simulink model "SF040A_MotVel"  (R2013b)
settings: Solver=FixedStepDiscrete  SolverMode=SingleTasking  StartTime=0.0  StopTime=1  FixedStep=6.25E-5  RelTol=1e-3
undefined symbols (not defined in the file or in its folder): ARCHGLBPRM_2MILLISEC_SEC_F32, ARCHGLBPRM_2PI_ULS_F32, ARCHGLBPRM_FLOATZEROTHD_ULS_F32, ARCHGLBPRM_PI_ULS_F32, BITMASK16BIT_CNT_U32, BUFSIZE_CNT_U08, BUFSIZECOMBD_CNT_U08, MOTAGMECHIDPTSIGTHD_ULS_U08, MOTVELMAXININVAL_CNT_U08, SECTOMICROSEC_ULS_F32, ZEROTISTAMP_MICROSEC_F32, ZEROTISTAMP_MICROSEC_U32
libraries: simulink x7, NxtrLim x2, FixdToFloat x1
(part 2 of 2)

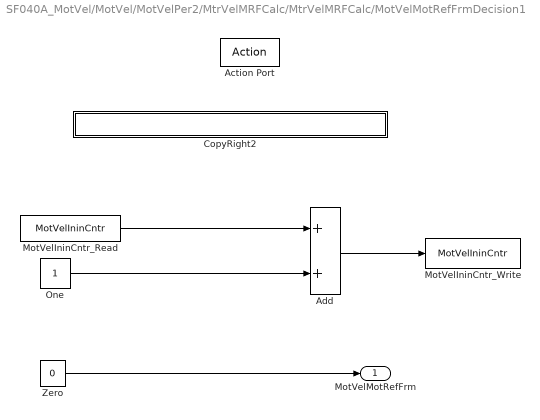
== system SF040A_MotVel/MotVel/MotVelPer2/MtrVelMRFCalc/MtrVelMRFCalc/MotVelMotRefFrmDecision1 ==
  Action Port : ActionPort  ActionType=then
  Add : Sum  OutDataTypeStr=Inherit: Inherit via back propagation
  CopyRight2 : Subsystem  Description=|  mask(Copyright Information){none=on}
      | Copyright info block.                                               
      |                                                                     
      | Place copyright information at the top of every subsystem in design.
      mask prompts: none "No parameters"
      mask help: Place copyright information at the top of every subsystem in design.
      mask Display:
      | NxtrConf = 'Nexteer Confidential';
      | 
      | sys = bdroot; %handle for the current model ("system")
      | first = get_param(sys,'Created');
      | first = first(end-3:end);  %year is last four digits
      | 
      | last = get_param(sys,'LastModifiedDate');
      | if isempty(last)
      |     last = datestr(now,'yyyy');
      | else
      |     last = last(end-3:end);
      | end
      | 
      | if strcmp(first,last)
      |     fprintf('%s -- Copyright %s Nexteer',NxtrConf,first)
      | else
      |     fprintf('%s -- %s%s- %s Nexteer',NxtrConf,char(169),first,last)
      | end
  MotVelIninCntr_Read : DataStoreRead  DataStoreName=MotVelIninCntr
  MotVelIninCntr_Write : DataStoreWrite  DataStoreName=MotVelIninCntr
  One : Constant  OutDataTypeStr=uint8
      settings: AttributesFormatString=%<OutDataTypeStr>
  Zero : Constant  Value=0  OutDataTypeStr=single
      settings: AttributesFormatString=%<OutDataTypeStr>
  MotVelMotRefFrm : Outport
  wires:
  Zero/1 -> MotVelMotRefFrm/1
  Add/1 -> MotVelIninCntr_Write/1
  One/1 -> Add/2
  MotVelIninCntr_Read/1 -> Add/1

== system SF040A_MotVel/MotVel/MotVelPer2/MtrVelMRFCalc/MtrVelMRFCalc/MotVelMotRefFrmDecision2 ==
  MotVelMrf : Inport
  Action Port : ActionPort  ActionType=else
  CopyRight2 : Subsystem  Description=|  mask(Copyright Information){none=on}
      | Copyright info block.                                               
      |                                                                     
      | Place copyright information at the top of every subsystem in design.
      mask prompts: none "No parameters"
      mask help: Place copyright information at the top of every subsystem in design.
      mask Display:
      | NxtrConf = 'Nexteer Confidential';
      | 
      | sys = bdroot; %handle for the current model ("system")
      | first = get_param(sys,'Created');
      | first = first(end-3:end);  %year is last four digits
      | 
      | last = get_param(sys,'LastModifiedDate');
      | if isempty(last)
      |     last = datestr(now,'yyyy');
      | else
      |     last = last(end-3:end);
      | end
      | 
      | if strcmp(first,last)
      |     fprintf('%s -- Copyright %s Nexteer',NxtrConf,first)
      | else
      |     fprintf('%s -- %s%s- %s Nexteer',NxtrConf,char(169),first,last)
      | end
  MotVelMotRefFrm : Outport
  wires:
  MotVelMrf/1 -> MotVelMotRefFrm/1

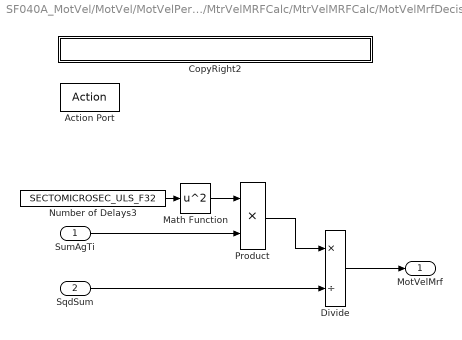
== system SF040A_MotVel/MotVel/MotVelPer2/MtrVelMRFCalc/MtrVelMRFCalc/MotVelMrfDecision1 ==
  SumAgTi : Inport
  SqdSum : Inport  Port=2
  Action Port : ActionPort  ActionType=then
  CopyRight2 : Subsystem  Description=|  mask(Copyright Information){none=on}
      | Copyright info block.                                               
      |                                                                     
      | Place copyright information at the top of every subsystem in design.
      mask prompts: none "No parameters"
      mask help: Place copyright information at the top of every subsystem in design.
      mask Display:
      | NxtrConf = 'Nexteer Confidential';
      | 
      | sys = bdroot; %handle for the current model ("system")
      | first = get_param(sys,'Created');
      | first = first(end-3:end);  %year is last four digits
      | 
      | last = get_param(sys,'LastModifiedDate');
      | if isempty(last)
      |     last = datestr(now,'yyyy');
      | else
      |     last = last(end-3:end);
      | end
      | 
      | if strcmp(first,last)
      |     fprintf('%s -- Copyright %s Nexteer',NxtrConf,first)
      | else
      |     fprintf('%s -- %s%s- %s Nexteer',NxtrConf,char(169),first,last)
      | end
  Divide : Product  Inputs=*/
  Math Function : Math  Operator=square  SaturateOnIntegerOverflow=on
  Number of Delays3 : Constant  Value=SECTOMICROSEC_ULS_F32
  Product : Product
  MotVelMrf : Outport
  wires:
  Number of Delays3/1 -> Math Function/1
  Math Function/1 -> Product/1
  SumAgTi/1 -> Product/2
  SqdSum/1 -> Divide/2
  Divide/1 -> MotVelMrf/1
  Product/1 -> Divide/1

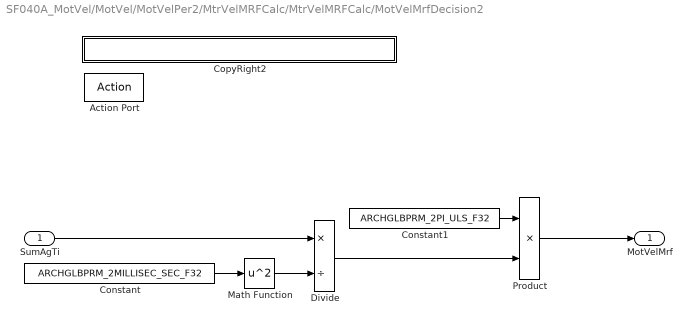
== system SF040A_MotVel/MotVel/MotVelPer2/MtrVelMRFCalc/MtrVelMRFCalc/MotVelMrfDecision2 ==
  SumAgTi : Inport
  Action Port : ActionPort  ActionType=else
  Constant : Constant  Value=ARCHGLBPRM_2MILLISEC_SEC_F32
  Constant1 : Constant  Value=ARCHGLBPRM_2PI_ULS_F32
  CopyRight2 : Subsystem  Description=|  mask(Copyright Information){none=on}
      | Copyright info block.                                               
      |                                                                     
      | Place copyright information at the top of every subsystem in design.
      mask prompts: none "No parameters"
      mask help: Place copyright information at the top of every subsystem in design.
      mask Display:
      | NxtrConf = 'Nexteer Confidential';
      | 
      | sys = bdroot; %handle for the current model ("system")
      | first = get_param(sys,'Created');
      | first = first(end-3:end);  %year is last four digits
      | 
      | last = get_param(sys,'LastModifiedDate');
      | if isempty(last)
      |     last = datestr(now,'yyyy');
      | else
      |     last = last(end-3:end);
      | end
      | 
      | if strcmp(first,last)
      |     fprintf('%s -- Copyright %s Nexteer',NxtrConf,first)
      | else
      |     fprintf('%s -- %s%s- %s Nexteer',NxtrConf,char(169),first,last)
      | end
  Divide : Product  Inputs=*/
  Math Function : Math  Operator=square  SaturateOnIntegerOverflow=on
  Product : Product
  MotVelMrf : Outport
  wires:
  SumAgTi/1 -> Divide/1
  Constant/1 -> Math Function/1
  Math Function/1 -> Divide/2
  Divide/1 -> Product/2
  Constant1/1 -> Product/1
  Product/1 -> MotVelMrf/1

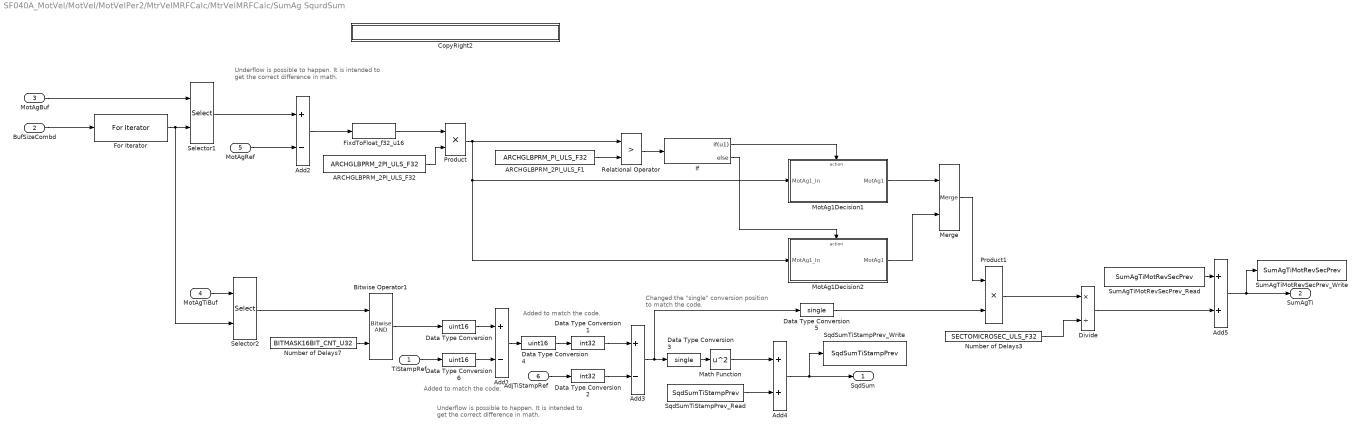
== system SF040A_MotVel/MotVel/MotVelPer2/MtrVelMRFCalc/MtrVelMRFCalc/SumAg SqurdSum ==
  note: Added to match the code.
  note: Underflow is possible to happen. It is intended
      | to get the correct difference in math.
  note: Underflow is possible to happen. It is intended
      | to get the correct difference in math.
  note: Changed the "single" conversion position
      |  to match the code.
  note: Added to match the code.
  TiStampRef : Inport
  BufSizeCombd : Inport  Port=2
  MotAgBuf : Inport  Port=3
  MotAgTiBuf : Inport  Port=4
  MotAgRef : Inport  Port=5
  AdjTiStampRef : Inport  Port=6
  ARCHGLBPRM_2PI_ULS_F1 : Constant  RequirementInfo="{'linktype_rmi_doors' '0000bab8 (/E-STEER Core/SubSystem Specifications/Application Functions/SF040A Motor Velocity)' '#SF040A_102' 'true' 'REQ:  SF040A_102' '' } %GIDa_2afc022e_23f4_4dbf_acb8_3ad7cf1d16c2"  Value=ARCHGLBPRM_PI_ULS_F32  OutDataTypeStr=single
  ARCHGLBPRM_2PI_ULS_F32 : Constant  Value=ARCHGLBPRM_2PI_ULS_F32  OutDataTypeStr=single
  Add1 : Sum  RequirementInfo="{'linktype_rmi_doors' '0000bab8 (/E-STEER Core/SubSystem Specifications/Application Functions/SF040A Motor Velocity)' '#SF040A_105' 'true' 'REQ:  SF040A_105' '' } %GIDa_0081e067_97a6_4f85_b01a_a6cee1fc1447"  Inputs=+-
  Add2 : Sum  RequirementInfo="{'linktype_rmi_doors' '0000bab8 (/E-STEER Core/SubSystem Specifications/Application Functions/SF040A Motor Velocity)' '#SF040A_105' 'true' 'REQ:  SF040A_105' '' } %GIDa_d704eb41_1352_4195_b5b6_a4582fe331e3"  Inputs=+-
  Add3 : Sum  RequirementInfo="{'linktype_rmi_doors' '0000bab8 (/E-STEER Core/SubSystem Specifications/Application Functions/SF040A Motor Velocity)' '#SF040A_105' 'true' 'REQ:  SF040A_105' '' } %GIDa_9c7c416f_a82a_4ea3_bcf9_a540842ea8b3"  Inputs=+-
  Add4 : Sum  RequirementInfo="{'linktype_rmi_doors' '0000bab8 (/E-STEER Core/SubSystem Specifications/Application Functions/SF040A Motor Velocity)' '#SF040A_105' 'true' 'REQ:  SF040A_105' '' } %GIDa_6bb91d2a_8ec1_41c7_a46f_9df07b2dccf6"
  Add5 : Sum  RequirementInfo="{'linktype_rmi_doors' '0000bab8 (/E-STEER Core/SubSystem Specifications/Application Functions/SF040A Motor Velocity)' '#SF040A_105' 'true' 'REQ:  SF040A_105' '' } %GIDa_7c248720_4236_4d8c_9ddf_d43ab10773e6"
  Bitwise Operator1 : simulink/Logic and Bit Operations/Bitwise Operator  RequirementInfo="{'linktype_rmi_doors' '0000bab8 (/E-STEER Core/SubSystem Specifications/Application Functions/SF040A Motor Velocity)' '#SF040A_105' 'true' 'REQ:  SF040A_105' '' } %GIDa_08a7f3b0_c0ea_42d7_9838_248064a04c32"  logicop=AND  UseBitMask=off  NumInputPorts=2  BitMask=bin2dec('')  BitMaskRealWorld=Stored Integer
  CopyRight2 : Subsystem  Description=|  mask(Copyright Information){none=on}
      | Copyright info block.                                               
      |                                                                     
      | Place copyright information at the top of every subsystem in design.
      mask prompts: none "No parameters"
      mask help: Place copyright information at the top of every subsystem in design.
      mask Display:
      | NxtrConf = 'Nexteer Confidential';
      | 
      | sys = bdroot; %handle for the current model ("system")
      | first = get_param(sys,'Created');
      | first = first(end-3:end);  %year is last four digits
      | 
      | last = get_param(sys,'LastModifiedDate');
      | if isempty(last)
      |     last = datestr(now,'yyyy');
      | else
      |     last = last(end-3:end);
      | end
      | 
      | if strcmp(first,last)
      |     fprintf('%s -- Copyright %s Nexteer',NxtrConf,first)
      | else
      |     fprintf('%s -- %s%s- %s Nexteer',NxtrConf,char(169),first,last)
      | end
  Data Type Conversion : DataTypeConversion  OutDataTypeStr=uint16
  Data Type Conversion1 : DataTypeConversion  OutDataTypeStr=int32
  Data Type Conversion2 : DataTypeConversion  OutDataTypeStr=int32
  Data Type Conversion3 : DataTypeConversion  OutDataTypeStr=single
  Data Type Conversion4 : DataTypeConversion  OutDataTypeStr=uint16
  Data Type Conversion5 : DataTypeConversion  OutDataTypeStr=single
  Data Type Conversion6 : DataTypeConversion  OutDataTypeStr=uint16
  Divide : Product  RequirementInfo="{'linktype_rmi_doors' '0000bab8 (/E-STEER Core/SubSystem Specifications/Application Functions/SF040A Motor Velocity)' '#SF040A_105' 'true' 'REQ:  SF040A_105' '' } %GIDa_88619ad8_fe51_49e2_b56e_2c73dbac99b3"  Inputs=*/
  FixdToFloat_f32_u16 : FixdToFloat/FixdToFloat_f32_u16  Param1=16
  For Iterator : ForIterator  RequirementInfo="{'linktype_rmi_doors' '0000bab8 (/E-STEER Core/SubSystem Specifications/Application Functions/SF040A Motor Velocity)' '#SF040A_105' 'true' 'REQ:  SF040A_105' '' } %GIDa_1101b510_28c4_4d50_b3ed_181c6f4250ed"  IterationSource=external  IndexMode=Zero-based  IterationVariableDataType=int8
  If : If  RequirementInfo="{'linktype_rmi_doors' '0000bab8 (/E-STEER Core/SubSystem Specifications/Application Functions/SF040A Motor Velocity)' '#SF040A_102' 'true' 'REQ:  SF040A_102' '' } %GIDa_4999496b_0fad_4199_9960_897316b736d2"  IfExpression=u1
  Math Function : Math  RequirementInfo="{'linktype_rmi_doors' '0000bab8 (/E-STEER Core/SubSystem Specifications/Application Functions/SF040A Motor Velocity)' '#SF040A_105' 'true' 'REQ:  SF040A_105' '' } %GIDa_7b59953f_2a67_4552_b232_78cd08fad8dd"  Operator=square  SaturateOnIntegerOverflow=on
  Merge : Merge  RequirementInfo="{'linktype_rmi_doors' '0000bab8 (/E-STEER Core/SubSystem Specifications/Application Functions/SF040A Motor Velocity)' '#SF040A_102' 'true' 'REQ:  SF040A_102' '' } %GIDa_56b2e5ce_0e8a_424c_bec4_d35ae6f6f09b"
  MotAg1Decision1 : Subsystem  RequirementInfo="{'linktype_rmi_doors' '0000bab8 (/E-STEER Core/SubSystem Specifications/Application Functions/SF040A Motor Velocity)' '#SF040A_102' 'true' 'REQ:  SF040A_102' '' } %GIDa_76cec83c_1dcb_497c_ae5b_3add9fa96ce7"  TreatAsAtomicUnit=on
  MotAg1Decision2 : Subsystem  RequirementInfo="{'linktype_rmi_doors' '0000bab8 (/E-STEER Core/SubSystem Specifications/Application Functions/SF040A Motor Velocity)' '#SF040A_102' 'true' 'REQ:  SF040A_102' '' } %GIDa_44da3dc5_3240_4e08_91f4_cd8830470459"  TreatAsAtomicUnit=on
  Number of Delays3 : Constant  Value=SECTOMICROSEC_ULS_F32
  Number of Delays7 : Constant  Value=BITMASK16BIT_CNT_U32
  Product : Product  RequirementInfo="{'linktype_rmi_doors' '0000bab8 (/E-STEER Core/SubSystem Specifications/Application Functions/SF040A Motor Velocity)' '#SF040A_105' 'true' 'REQ:  SF040A_105' '' } %GIDa_6db179b0_8f89_47f3_9585_05f2d8a76b9a"
  Product1 : Product  RequirementInfo="{'linktype_rmi_doors' '0000bab8 (/E-STEER Core/SubSystem Specifications/Application Functions/SF040A Motor Velocity)' '#SF040A_105' 'true' 'REQ:  SF040A_105' '' } %GIDa_d1ae0e83_581f_412a_bee8_7ff3a18431f5"  RndMeth=Zero
  Relational Operator : RelationalOperator  RequirementInfo="{'linktype_rmi_doors' '0000bab8 (/E-STEER Core/SubSystem Specifications/Application Functions/SF040A Motor Velocity)' '#SF040A_102' 'true' 'REQ:  SF040A_102' '' } %GIDa_f7804aa1_faa5_4ed0_bd03_9321eff60666"  Operator=>  OutDataTypeStr=boolean
  Selector1 : Selector  RequirementInfo="{'linktype_rmi_doors' '0000bab8 (/E-STEER Core/SubSystem Specifications/Application Functions/SF040A Motor Velocity)' '#SF040A_105' 'true' 'REQ:  SF040A_105' '' } %GIDa_2fe4299a_f1d6_4ee5_8210_6d1d6d94a0c2"  IndexMode=Zero-based  InputPortWidth=16  IndexOptions=Index vector (port)  Indices=[1 3]  OutputSizes=1
  Selector2 : Selector  RequirementInfo="{'linktype_rmi_doors' '0000bab8 (/E-STEER Core/SubSystem Specifications/Application Functions/SF040A Motor Velocity)' '#SF040A_105' 'true' 'REQ:  SF040A_105' '' } %GIDa_cda2faf0_844d_468b_a74f_a0942cc6f198"  IndexMode=Zero-based  InputPortWidth=16  IndexOptions=Index vector (port)  Indices=[1 3]  OutputSizes=1
  SqdSumTiStampPrev_Read : DataStoreRead  DataStoreName=SqdSumTiStampPrev
  SqdSumTiStampPrev_Write : DataStoreWrite  DataStoreName=SqdSumTiStampPrev
  SumAgTiMotRevSecPrev_Read : DataStoreRead  DataStoreName=SumAgTiMotRevSecPrev
  SumAgTiMotRevSecPrev_Write : DataStoreWrite  DataStoreName=SumAgTiMotRevSecPrev
  SqdSum : Outport
  SumAgTi : Outport  Port=2
  wires:
  ARCHGLBPRM_2PI_ULS_F1/1 -> Relational Operator/2
  MotAgBuf/1 -> Selector1/1
  BufSizeCombd/1 -> For Iterator/1
  For Iterator/1 -> Selector2/2, Selector1/2
  Selector1/1 -> Add2/1
  MotAgRef/1 -> Add2/2
  Add2/1 -> FixdToFloat_f32_u16/1
  ARCHGLBPRM_2PI_ULS_F32/1 -> Product/2
  FixdToFloat_f32_u16/1 -> Product/1
  Relational Operator/1 -> If/1
  If/1 -> MotAg1Decision1/Action
  If/2 -> MotAg1Decision2/Action
  MotAg1Decision2/1(MotAg1) -> Merge/2
  MotAg1Decision1/1(MotAg1) -> Merge/1
  MotAgTiBuf/1 -> Selector2/1
  Number of Delays7/1 -> Bitwise Operator1/2
  Selector2/1 -> Bitwise Operator1/1
  Bitwise Operator1/1 -> Data Type Conversion/1
  Data Type Conversion/1 -> Add1/1
  TiStampRef/1 -> Data Type Conversion6/1
  Add1/1 -> Data Type Conversion4/1
  Data Type Conversion1/1 -> Add3/1
  AdjTiStampRef/1 -> Data Type Conversion2/1
  Data Type Conversion2/1 -> Add3/2
  Add3/1 -> Data Type Conversion5/1, Data Type Conversion3/1
  Math Function/1 -> Add4/1
  SqdSumTiStampPrev_Read/1 -> Add4/2
  Add4/1 -> SqdSumTiStampPrev_Write/1, SqdSum/1
  Merge/1 -> Product1/1
  Product1/1 -> Divide/1
  Number of Delays3/1 -> Divide/2
  SumAgTiMotRevSecPrev_Read/1 -> Add5/1
  Add5/1 -> SumAgTi/1, SumAgTiMotRevSecPrev_Write/1
  Product/1 -> Relational Operator/1, MotAg1Decision2/1(MotAg1_In), MotAg1Decision1/1(MotAg1_In)
  Divide/1 -> Add5/2
  Data Type Conversion3/1 -> Math Function/1
  Data Type Conversion4/1 -> Data Type Conversion1/1
  Data Type Conversion5/1 -> Product1/2
  Data Type Conversion6/1 -> Add1/2

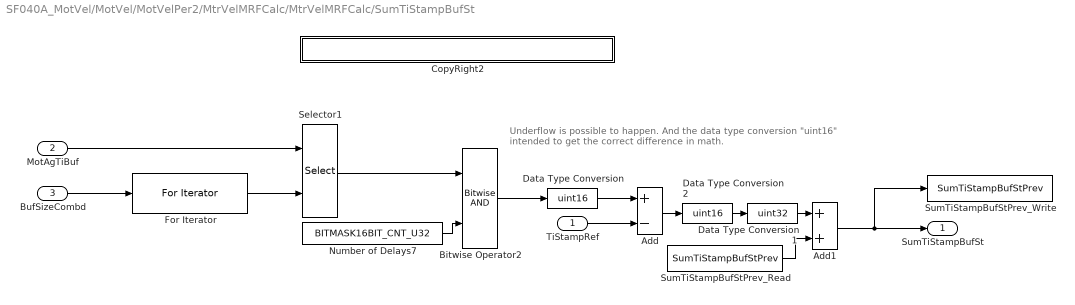
== system SF040A_MotVel/MotVel/MotVelPer2/MtrVelMRFCalc/MtrVelMRFCalc/SumTiStampBufSt ==
  note: Underflow is possible to happen. And the data type conversion "uint16"
      | intended to get the correct difference in math.
  TiStampRef : Inport
  MotAgTiBuf : Inport  Port=2
  BufSizeCombd : Inport  Port=3
  Add : Sum  RequirementInfo="{'linktype_rmi_doors' '0000bab8 (/E-STEER Core/SubSystem Specifications/Application Functions/SF040A Motor Velocity)' '#SF040A_103' 'true' 'REQ:  SF040A_103' '' } %GIDa_a2f324f7_36c5_4832_8266_b4ce5dbf6b9c"  Inputs=+-
  Add1 : Sum  RequirementInfo="{'linktype_rmi_doors' '0000bab8 (/E-STEER Core/SubSystem Specifications/Application Functions/SF040A Motor Velocity)' '#SF040A_103' 'true' 'REQ:  SF040A_103' '' } %GIDa_5290e7ed_18c1_402a_8a7a_c56c04379a42"
  Bitwise Operator2 : simulink/Logic and Bit Operations/Bitwise Operator  RequirementInfo="{'linktype_rmi_doors' '0000bab8 (/E-STEER Core/SubSystem Specifications/Application Functions/SF040A Motor Velocity)' '#SF040A_103' 'true' 'REQ:  SF040A_103' '' } %GIDa_50ad2c73_35f4_49be_8ca7_7f3f5b534c0f"  logicop=AND  UseBitMask=off  NumInputPorts=2  BitMask=bin2dec('')  BitMaskRealWorld=Stored Integer
  CopyRight2 : Subsystem  Description=|  mask(Copyright Information){none=on}
      | Copyright info block.                                               
      |                                                                     
      | Place copyright information at the top of every subsystem in design.
      mask prompts: none "No parameters"
      mask help: Place copyright information at the top of every subsystem in design.
      mask Display:
      | NxtrConf = 'Nexteer Confidential';
      | 
      | sys = bdroot; %handle for the current model ("system")
      | first = get_param(sys,'Created');
      | first = first(end-3:end);  %year is last four digits
      | 
      | last = get_param(sys,'LastModifiedDate');
      | if isempty(last)
      |     last = datestr(now,'yyyy');
      | else
      |     last = last(end-3:end);
      | end
      | 
      | if strcmp(first,last)
      |     fprintf('%s -- Copyright %s Nexteer',NxtrConf,first)
      | else
      |     fprintf('%s -- %s%s- %s Nexteer',NxtrConf,char(169),first,last)
      | end
  Data Type Conversion : DataTypeConversion  OutDataTypeStr=uint16
  Data Type Conversion1 : DataTypeConversion  OutDataTypeStr=uint32
  Data Type Conversion2 : DataTypeConversion  OutDataTypeStr=uint16
  For Iterator : ForIterator  RequirementInfo="{'linktype_rmi_doors' '0000bab8 (/E-STEER Core/SubSystem Specifications/Application Functions/SF040A Motor Velocity)' '#SF040A_103' 'true' 'REQ:  SF040A_103' '' } %GIDa_f36e4621_1bb4_45cf_b681_c1302a74f80e"  IterationSource=external  IndexMode=Zero-based  IterationVariableDataType=int8
  Number of Delays7 : Constant  Value=BITMASK16BIT_CNT_U32
  Selector1 : Selector  RequirementInfo="{'linktype_rmi_doors' '0000bab8 (/E-STEER Core/SubSystem Specifications/Application Functions/SF040A Motor Velocity)' '#SF040A_103' 'true' 'REQ:  SF040A_103' '' } %GIDa_b3146c9e_032e_4c7d_b57c_054ca58eb257"  IndexMode=Zero-based  InputPortWidth=16  IndexOptions=Index vector (port)  Indices=[1 3]  OutputSizes=1
  SumTiStampBufStPrev_Read : DataStoreRead  DataStoreName=SumTiStampBufStPrev
  SumTiStampBufStPrev_Write : DataStoreWrite  DataStoreName=SumTiStampBufStPrev
  SumTiStampBufSt : Outport
  wires:
  BufSizeCombd/1 -> For Iterator/1
  For Iterator/1 -> Selector1/2
  MotAgTiBuf/1 -> Selector1/1
  Selector1/1 -> Bitwise Operator2/1
  Number of Delays7/1 -> Bitwise Operator2/2
  Bitwise Operator2/1 -> Data Type Conversion/1
  TiStampRef/1 -> Add/2
  Data Type Conversion/1 -> Add/1
  Add/1 -> Data Type Conversion2/1
  Data Type Conversion1/1 -> Add1/1
  SumTiStampBufStPrev_Read/1 -> Add1/2
  Add1/1 -> SumTiStampBufStPrev_Write/1, SumTiStampBufSt/1
  Data Type Conversion2/1 -> Data Type Conversion1/1

== system SF040A_MotVel/MotVel/MotVelPer2/MtrVelMRFCalc/MtrVelMRFCalc/MotVelMotRefFrmDecision1/CopyRight2 ==

== system SF040A_MotVel/MotVel/MotVelPer2/MtrVelMRFCalc/MtrVelMRFCalc/MotVelMotRefFrmDecision2/CopyRight2 ==

== system SF040A_MotVel/MotVel/MotVelPer2/MtrVelMRFCalc/MtrVelMRFCalc/MotVelMrfDecision1/CopyRight2 ==

== system SF040A_MotVel/MotVel/MotVelPer2/MtrVelMRFCalc/MtrVelMRFCalc/MotVelMrfDecision2/CopyRight2 ==

== system SF040A_MotVel/MotVel/MotVelPer2/MtrVelMRFCalc/MtrVelMRFCalc/SumAg SqurdSum/CopyRight2 ==

== system SF040A_MotVel/MotVel/MotVelPer2/MtrVelMRFCalc/MtrVelMRFCalc/SumAg SqurdSum/MotAg1Decision1 ==
  MotAg1_In : Inport
  Action Port : ActionPort  ActionType=then
  Add : Sum  Inputs=+-
  Constant : Constant  Value=ARCHGLBPRM_2PI_ULS_F32  OutDataTypeStr=single
  CopyRight2 : Subsystem  Description=|  mask(Copyright Information){none=on}
      | Copyright info block.                                               
      |                                                                     
      | Place copyright information at the top of every subsystem in design.
      mask prompts: none "No parameters"
      mask help: Place copyright information at the top of every subsystem in design.
      mask Display:
      | NxtrConf = 'Nexteer Confidential';
      | 
      | sys = bdroot; %handle for the current model ("system")
      | first = get_param(sys,'Created');
      | first = first(end-3:end);  %year is last four digits
      | 
      | last = get_param(sys,'LastModifiedDate');
      | if isempty(last)
      |     last = datestr(now,'yyyy');
      | else
      |     last = last(end-3:end);
      | end
      | 
      | if strcmp(first,last)
      |     fprintf('%s -- Copyright %s Nexteer',NxtrConf,first)
      | else
      |     fprintf('%s -- %s%s- %s Nexteer',NxtrConf,char(169),first,last)
      | end
  MotAg1 : Outport
  wires:
  Constant/1 -> Add/2
  MotAg1_In/1 -> Add/1
  Add/1 -> MotAg1/1

== system SF040A_MotVel/MotVel/MotVelPer2/MtrVelMRFCalc/MtrVelMRFCalc/SumAg SqurdSum/MotAg1Decision2 ==
  MotAg1_In : Inport
  Action Port : ActionPort  ActionType=else
  CopyRight2 : Subsystem  Description=|  mask(Copyright Information){none=on}
      | Copyright info block.                                               
      |                                                                     
      | Place copyright information at the top of every subsystem in design.
      mask prompts: none "No parameters"
      mask help: Place copyright information at the top of every subsystem in design.
      mask Display:
      | NxtrConf = 'Nexteer Confidential';
      | 
      | sys = bdroot; %handle for the current model ("system")
      | first = get_param(sys,'Created');
      | first = first(end-3:end);  %year is last four digits
      | 
      | last = get_param(sys,'LastModifiedDate');
      | if isempty(last)
      |     last = datestr(now,'yyyy');
      | else
      |     last = last(end-3:end);
      | end
      | 
      | if strcmp(first,last)
      |     fprintf('%s -- Copyright %s Nexteer',NxtrConf,first)
      | else
      |     fprintf('%s -- %s%s- %s Nexteer',NxtrConf,char(169),first,last)
      | end
  MotAg1 : Outport
  wires:
  MotAg1_In/1 -> MotAg1/1

== system SF040A_MotVel/MotVel/MotVelPer2/MtrVelMRFCalc/MtrVelMRFCalc/SumTiStampBufSt/CopyRight2 ==

== system SF040A_MotVel/MotVel/MotVelPer2/MtrVelMRFCalc/MtrVelMRFCalc/SumAg SqurdSum/MotAg1Decision1/CopyRight2 ==

== system SF040A_MotVel/MotVel/MotVelPer2/MtrVelMRFCalc/MtrVelMRFCalc/SumAg SqurdSum/MotAg1Decision2/CopyRight2 ==
